simulink model "kadai41"  (R2021b)
settings: Solver=VariableStepAuto  StartTime=0.0  StopTime=20  MaxStep=0.001  RelTol=1e-3
settings Model: NumberOfSteps=400000  Creator=is221042  LastModifiedBy=tomotomo

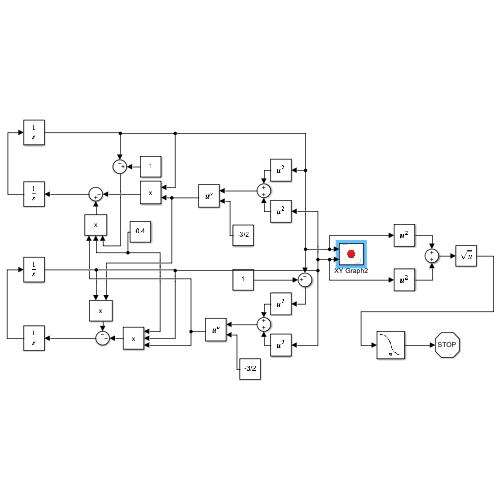
[thumbnail: Simulink's stored preview of the top-level diagram]
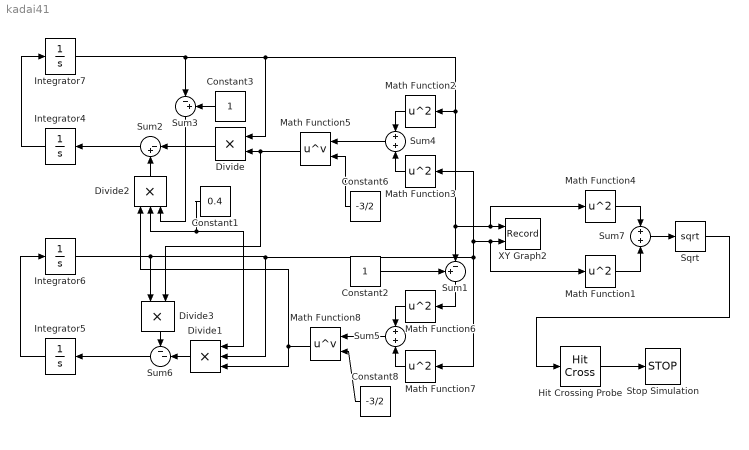
== system kadai41 ==
  Constant1 : Constant  Value=0.4
  Constant2 : Constant
  Constant3 : Constant
  Constant6 : Constant  Value=-3/2
  Constant8 : Constant  Value=-3/2
  Divide : Product  Inputs=**
  Divide1 : Product  Inputs=***
  Divide2 : Product  Inputs=***
  Divide3 : Product  Inputs=**
  Hit Crossing Probe : HitCross  HitCrossingOffset=0.2  HitCrossingDirection=falling
  Integrator4 : Integrator  InitialCondition=-0.399
  Integrator5 : Integrator  InitialCondition=3.0
  Integrator6 : Integrator  InitialCondition=0.0
  Integrator7 : Integrator  InitialCondition=-0.2
  Math Function{1..4,6..7} (6 alike) : Math  Operator=square  SaturateOnIntegerOverflow=on
  Math Function5 : Math  Operator=pow  SaturateOnIntegerOverflow=on
  Math Function8 : Math  Operator=pow  SaturateOnIntegerOverflow=on
  Sqrt : Sqrt  SaturateOnIntegerOverflow=on
  Stop Simulation : Stop
  Sum1 : Sum  Inputs=+-|
  Sum2 : Sum  Inputs=|-+
  Sum3 : Sum  Inputs=|-+
  Sum4 : Sum  Inputs=+|+
  Sum5 : Sum  Inputs=+|+
  Sum6 : Sum  Inputs=--|
  Sum7 : Sum  Inputs=+|+
  XY Graph2 : Record  FileSettingsInternal="{\"entries\":[{\"content\":{\"excelSettings\":{\"content\":{},\"type\":\"Streamout.ExcelSettings\"}},\"type\":\"Streamout.FileSettingStorage\",\"uuid\":\"65a9beba-e992-4559-a012-979efefdfe69\"}],\"packageUris\":[\"http://schema.mathworks.com/mf0/streamout_blocks/R2020a\"],\"version\":\"1.0\"}"  Layout=[1 1]  SignalsInternal="{\"entries\":[{\"content\":{\"signals\":[{\"content\":{\"blockPath\":[\"kadai41/XY Graph2\"],\"channel\":[],\"dimensions\":[1],\"domain\":\"kadai41/XY Graph2\",\"lineColor\":\"#a2142f\",\"plots\":[1],\"port\":1,\"sid\":[\"\"],\"signalID\":216,\"signalName\":\"Integrator7\"},\"type\":\"RecordBlkView.Signal\",\"uuid\":\"7f3f7b70-7f27-4802-9ca8-f4657650877a\"},{\"content\":{\"blockPath\":[\"kadai41/XY Graph2\"],\"channel\":[],\"dimensions\":[1],\"domain\":\"kadai41/XY Graph2\",\"lineColor\":\"#139fff\",\"plots\":[1],\"port\":2,\"sid\":[\"\"],\"signalID\":220,\"signalName\":\"Integrator6\"},\"type\":\"RecordBlkView.Signal\",\"uuid\":\"90ab1d30-1ff7-477d-a616-8f66439350a2\"}]},\"type\":\"RecordBlkView.InputSignals\",\"uuid\":\"cc232157-5148-4191-8caa-3107282610ac\"}],\"packageUris\":[\"http://schema.mathworks.com/mf0/streamout_blocks/R2020a\"],\"version\":\"1.0\"}"  VisualizationBindings="{\"xyplotplugin\":{\"info\":[{\"series\":[{\"bindingParametersList\":[{\"parameter\":\"X-Axis\",\"signalID\":216,\"signalName\":\"Integrator7\"},{\"parameter\":\"Y-Axis\",\"signalID\":220,\"signalName\":\"Integrator6\"}],\"seriesID\":38814}],\"subplotID\":1}]}}"  CompatibilityTag=XY
  wires:
  Integrator7/1 -> Sum3/1, Divide/1, Math Function4/1, XY Graph2/1, Sum1/2, Math Function2/1
  Sum5/1 -> Math Function8/1
  Integrator6/1 -> Divide3/1, Divide1/2, Math Function1/1, XY Graph2/2, Math Function3/1, Math Function7/1
  Math Function6/1 -> Sum5/1
  Math Function7/1 -> Sum5/2
  Constant6/1 -> Math Function5/2
  Constant8/1 -> Math Function8/2
  Sum4/1 -> Math Function5/1
  Math Function8/1 -> Divide1/3, Divide2/1
  Math Function3/1 -> Sum4/2
  Math Function5/1 -> Divide3/2, Divide/2
  Integrator4/1 -> Integrator7/1
  Math Function2/1 -> Sum4/1
  Integrator5/1 -> Integrator6/1
  Constant2/1 -> Sum1/1
  Sum1/1 -> Math Function6/1
  Divide/1 -> Sum2/1
  Divide2/1 -> Sum2/2
  Sum3/1 -> Divide2/3
  Constant3/1 -> Sum3/2
  Constant1/1 -> Divide1/1, Divide2/2
  Sum2/1 -> Integrator4/1
  Divide3/1 -> Sum6/1
  Divide1/1 -> Sum6/2
  Sum6/1 -> Integrator5/1
  Sum7/1 -> Sqrt/1
  Math Function4/1 -> Sum7/1
  Math Function1/1 -> Sum7/2
  Sqrt/1 -> Hit Crossing Probe/1
  Hit Crossing Probe/1 -> Stop Simulation/1
